simulink library "csu_tfl_thruster_forces_mtv_lib"  (R2014b)
settings: Solver=ode45  StartTime=0.0  StopTime=10.0  RelTol=1e-3
libraries: util_thruster_lib x12, util_info_lib x1
settings Model: Creator=Nilesh  LastModifiedBy=mstewart

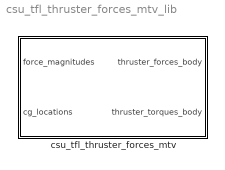
== system csu_tfl_thruster_forces_mtv_lib ==
  csu_tfl_thruster_forces_mtv : Subsystem

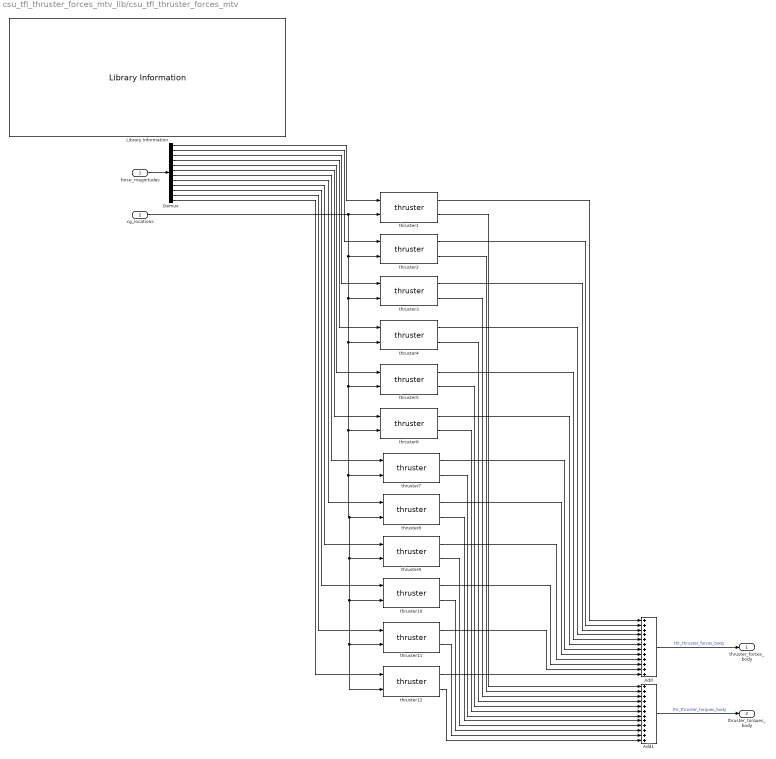
== system csu_tfl_thruster_forces_mtv_lib/csu_tfl_thruster_forces_mtv ==
  force_magnitudes : Inport
  cg_locations : Inport  Port=2
  Add : Sum  Inputs=++++++++++++
  Add1 : Sum  Inputs=++++++++++++
  Demux : Demux  Outputs=12
  Library Information : util_info_lib/Library Information  owner='escrane'
  thruster1 : util_thruster_lib/thruster  Thruster_Position=tfl_thruster1_position  Thruster_Orientation=tfl_thruster1_orientation
  thruster10 : util_thruster_lib/thruster  Thruster_Position=tfl_thruster10_position  Thruster_Orientation=tfl_thruster10_orientation
  thruster11 : util_thruster_lib/thruster  Thruster_Position=tfl_thruster11_position  Thruster_Orientation=tfl_thruster11_orientation
  thruster12 : util_thruster_lib/thruster  Thruster_Position=tfl_thruster12_position  Thruster_Orientation=tfl_thruster12_orientation
  thruster2 : util_thruster_lib/thruster  Thruster_Position=tfl_thruster2_position  Thruster_Orientation=tfl_thruster2_orientation
  thruster3 : util_thruster_lib/thruster  Thruster_Position=tfl_thruster3_position  Thruster_Orientation=tfl_thruster3_orientation
  thruster4 : util_thruster_lib/thruster  Thruster_Position=tfl_thruster4_position  Thruster_Orientation=tfl_thruster4_orientation
  thruster5 : util_thruster_lib/thruster  Thruster_Position=tfl_thruster5_position  Thruster_Orientation=tfl_thruster5_orientation
  thruster6 : util_thruster_lib/thruster  Thruster_Position=tfl_thruster6_position  Thruster_Orientation=tfl_thruster6_orientation
  thruster7 : util_thruster_lib/thruster  Thruster_Position=tfl_thruster7_position  Thruster_Orientation=tfl_thruster7_orientation
  thruster8 : util_thruster_lib/thruster  Thruster_Position=tfl_thruster8_position  Thruster_Orientation=tfl_thruster8_orientation
  thruster9 : util_thruster_lib/thruster  Thruster_Position=tfl_thruster9_position  Thruster_Orientation=tfl_thruster9_orientation
  thruster_forces_body : Outport
  thruster_torques_body : Outport  Port=2
  wires:
  cg_locations/1 -> thruster7/2, thruster12/2, thruster11/2, thruster10/2, thruster9/2, thruster8/2, thruster6/2, thruster5/2, thruster4/2, thruster3/2, thruster2/2, thruster1/2
  force_magnitudes/1 -> Demux/1
  Add1/1 -> thruster_torques_body/1  "thr_thruster_torques_body"
  thruster1/1 -> Add/1
  thruster2/1 -> Add/2
  thruster3/1 -> Add/3
  Demux/1 -> thruster1/1
  Demux/2 -> thruster2/1
  Demux/3 -> thruster3/1
  Demux/4 -> thruster4/1
  Demux/5 -> thruster5/1
  Demux/6 -> thruster6/1
  Demux/7 -> thruster7/1
  thruster1/2 -> Add1/1
  thruster2/2 -> Add1/2
  thruster3/2 -> Add1/3
  thruster4/2 -> Add1/4
  thruster5/2 -> Add1/5
  thruster6/2 -> Add1/6
  thruster7/2 -> Add1/7
  Add/1 -> thruster_forces_body/1  "thr_thruster_forces_body"
  Demux/8 -> thruster8/1
  Demux/9 -> thruster9/1
  Demux/10 -> thruster10/1
  Demux/11 -> thruster11/1
  Demux/12 -> thruster12/1
  thruster4/1 -> Add/4
  thruster5/1 -> Add/5
  thruster6/1 -> Add/6
  thruster7/1 -> Add/7
  thruster8/1 -> Add/8
  thruster9/1 -> Add/9
  thruster10/1 -> Add/10
  thruster11/1 -> Add/11
  thruster12/1 -> Add/12
  thruster8/2 -> Add1/8
  thruster9/2 -> Add1/9
  thruster10/2 -> Add1/10
  thruster11/2 -> Add1/11
  thruster12/2 -> Add1/12
